simulink model "Unbatch_Model"  (R2024b)
settings: Solver=VariableStepAuto  StartTime=0.0  StopTime=10.0  RelTol=1e-3
libraries: NSA_DEVS_LOGISTICS x3, NSA_DEVS_SOURCES x2, NSA_DEVS_SINKS x1
settings Model: Creator=david  LastModifiedBy=peter
settings RTWCC: GPUComputeCapability=3.5

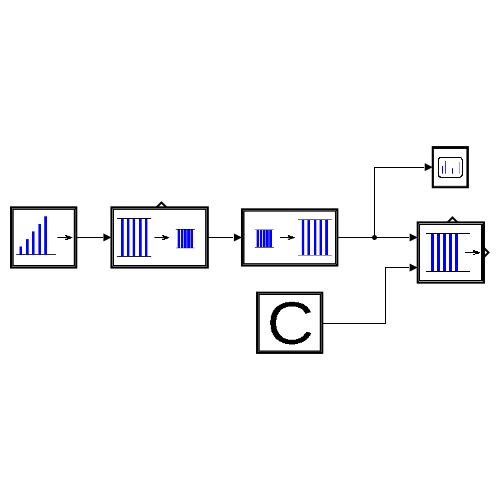
[thumbnail: Simulink's stored preview of the top-level diagram]
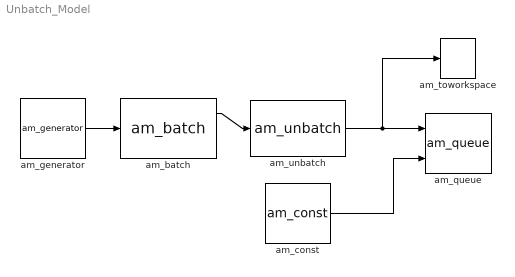
== system Unbatch_Model ==
  am_batch : NSA_DEVS_LOGISTICS/am_batch  N=10  tau=[0,1]  debug=0
      settings: SourceProductName=Logistics
  am_const : NSA_DEVS_SOURCES/am_const  value=true  sendTime=[0,1]  tau=[0,1]  debug=0
      settings: SourceProductName=Sources
  am_generator : NSA_DEVS_SOURCES/am_generator  tG=1  n0=0  nG=inf  tD=[0,2]  debug=0
      settings: SourceProductName=Sources
  am_queue : NSA_DEVS_LOGISTICS/am_queue  tD=[0,1]  tau=[0,1]  debug=0
      settings: SourceProductName=Logistics
  am_toworkspace : NSA_DEVS_SINKS/am_toworkspace  varname="\"out\""  t0=0  format="\"vector\""  tau=[0,0.5]  debug=0
      settings: SourceProductName=Sinks
  am_unbatch : NSA_DEVS_LOGISTICS/am_unbatch  tD=[0,1]  tau=[0,2]  debug=0
      settings: SourceProductName=Logistics
  wires:
  am_generator/1 -> am_batch/1
  am_batch/1 -> am_unbatch/1
  am_unbatch/1 -> am_toworkspace/1, am_queue/1
  am_const/1 -> am_queue/2
